simulink model "prospettiva"  (Simulink 7.6)
settings: Solver=FixedStepDiscrete  StartTime=0.0  StopTime=inf  RelTol=1e-3
undefined symbols (not defined in the file or in its folder): gray, none, Rec, SDTV, videoinput
libraries: vipconversions x2, vipsnks x2, imaqlib x1
settings Model: Creator=don  LastModifiedBy=seb  ExtModeAutoUpdateStatusClock=off
settings DataIOCC: LimitDataPoints=off  SaveOutput=off  SaveTime=off  SignalLoggingName=sigsOut
settings OptimizationCC: InitFltsAndDblsToZero=on  SimCompilerOptimization=On
settings DebuggingCC: CheckExecutionContextPreStartOutputMsg=on  CheckExecutionContextRuntimeOutputMsg=on  SignalResolutionControl=TryResolveAllWithWarning  SolverPrmCheckMsg=none  MultiTaskDSMMsg=warning  MultiTaskCondExecSysMsg=none  SigSpecEnsureSampleTimeMsg=none  StrictBusMsg=None
settings HardwareCC: TargetEndianess=LittleEndian  TargetHWDeviceType=Generic->MATLAB Host Computer  ProdEqTarget=off
settings RTWCC: IncludeERTFirstTime=on  RTWCompilerOptimization=On
settings GRTTargetCC: TargetFcnLib=ansi_tfl_tmw_new.mat

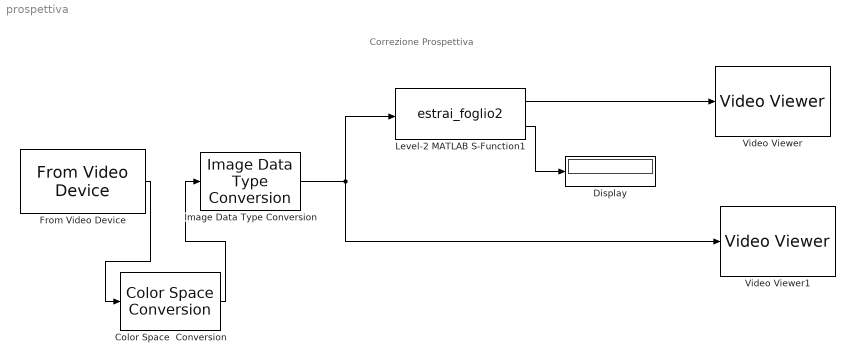
== system prospettiva ==
  note: Correzione Prospettiva
  Color Space  Conversion : vipconversions/Color Space  Conversion  conversion=Obsolete  conversionActive=Y'CbCr to R'G'B'  wp_str=D65  rec=Rec. 601 (SDTV)  sys=1125/60/2:1  imagePorts=One multidimensional signal
  Display : Display
  From Video Device : imaqlib/From Video Device  DialogController=imaqcreatedialog  DialogControllerArgs=DataTag1  DeviceMenu=winvideo 1 (Periferica video USB)  Device=winvideo 1 (Periferica video USB)  ObjConstructor=videoinput('winvideo', 1)  VideoFormatMenu=YUY2_1280x1024  VideoFormat=YUY2_1280x1024  VideoSource=input1  ROIPosition=[0 0 1024 1280]  EnableHWTrigger=off  TriggerConfiguration=none/none  SampleTime=1/30  OutputPortsMode=One multidimensional signal  DataType=double  CanDoHWTrigger=no  ReturnedColorSpace=YCbCr  BlockHandle=6.0012  ROIWidth=1280  ROIHeight=1024  ROIColumn=0  ROIRow=0  EngXMLPath=C:\Programmi\MATLAB\R2010b\toolbox\imaq\imaq\private  DevXMLPath=C:\Programmi\MATLAB\R2010b\toolbox\imaq\imaqadaptors\win32  EngLibPath=C:\Programmi\MATLAB\R2010b\toolbox\imaq\imaqblks\imaqmex\win32
  Image Data Type Conversion : vipconversions/Image Data Type Conversion  outDT=uint8  isSigned=on  wordLen=16  numFracBits=0
  Level-2 MATLAB S-Function1 : M-S-Function  FunctionName=estrai_foglio2  Parameters=3
  Video Viewer : vipsnks/Video Viewer  DialogControllerArgs=DataTag3  inputType=Obsolete7b  imagePorts=One multidimensional signal  useColorMap=off  colormapValue=gray(256)  specRange=off  minInputVal=0  maxInputVal=255  FigPos=[40 707 710 583]  AxisZoom=on  trueSizedOnce=off  OpenAtMdlStart=on
  Video Viewer1 : vipsnks/Video Viewer  DialogControllerArgs=DataTag5  inputType=Obsolete7b  imagePorts=One multidimensional signal  useColorMap=off  colormapValue=gray(256)  specRange=off  minInputVal=0  maxInputVal=255  FigPos=[563 967 666 607]  AxisZoom=on  trueSizedOnce=off  OpenAtMdlStart=on
  wires:
  Image Data Type Conversion/1 -> Level-2 MATLAB S-Function1/1, Video Viewer1/1
  Level-2 MATLAB S-Function1/1 -> Video Viewer/1
  Level-2 MATLAB S-Function1/2 -> Display/1
  From Video Device/1 -> Color Space  Conversion/1
  Color Space  Conversion/1 -> Image Data Type Conversion/1
